simulink model "kalman_picar"  (R2021b)
settings: Solver=VariableStepAuto  StartTime=0.0  StopTime=100  RelTol=1e-3
values from neighbouring files (symbols this model uses):
  A_kf = [1 delta_t;0 1]    [picar_kalman.m]
  acc_x = 2    [picar_kalman.m]
  b_kf = [delta_t^2/2; delta_t]    [picar_kalman.m]
  f_s = 100    [picar_kalman.m]
  sensor_cov = cov(transpose(stationary(acc_x:gyro_z,:)))    [picar_kalman.m]
  sensor_mean = mean(stationary(acc_x:gyro_z,:),2)    [picar_kalman.m]
undefined symbols (not defined in the file or in its folder): Discrete, Time
libraries: ctrlSharedLib x1
settings Model: Creator=willwu  LastModifiedBy=willwu

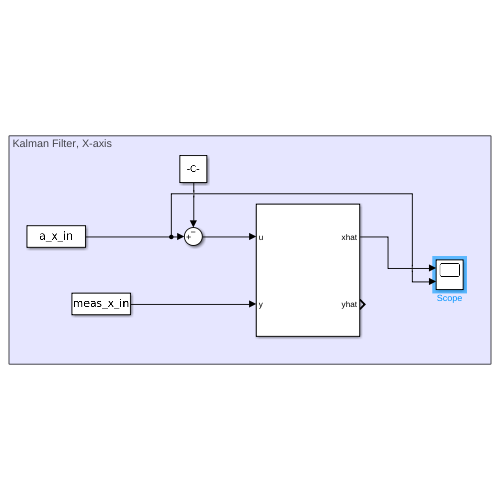
[thumbnail: Simulink's stored preview of the top-level diagram]
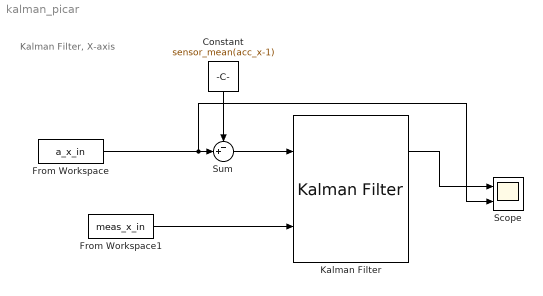
== system kalman_picar ==
  note: Kalman Filter, X-axis
  Constant : Constant  Value=sensor_mean(acc_x-1)
  From Workspace : FromWorkspace  VariableName=a_x_in  SampleTime=1/f_s
  From Workspace1 : FromWorkspace  VariableName=meas_x_in  SampleTime=1/f_s
  Kalman Filter : ctrlSharedLib/Kalman Filter  TimeDomain=Discrete-Time  UseCurrentEstimator=on  ModelSource=Individual A, B, C, D matrices  ModelSourceVariable=ss(0.95,1,1,0,1)  A=A_kf  B=b_kf  C=[1 0]  D=0  NumberOfStates=1  NumberOfInputs=1  NumberOfOutputs=1  InitialEstimateSource=Dialog  X0=0  P0=10  UseK=off  UseGH=off  NumberOfProcessNoiseInputs=1  G=1  TimeInvariantG=on  H=0  TimeInvariantH=on  Q=sensor_cov(1)  TimeInvariantQ=on  R=0.01  TimeInvariantR=on  N=0  TimeInvariantN=on  AddInputPort=on  AddEnablePort=off  OutputEstimatedY=on  OutputP=off  Ts=-1
  Scope : Scope  NumInputPorts=2
  Sum : Sum  Inputs=-+|
  wires:
  From Workspace/1 -> Scope/2, Sum/2
  Sum/1 -> Kalman Filter/1
  Constant/1 -> Sum/1
  Kalman Filter/1 -> Scope/1
  From Workspace1/1 -> Kalman Filter/2
